simulink model "untitled"  (R2017b)
settings: Solver=VariableStepAuto  StartTime=0.0  StopTime=10.0  RelTol=1e-3
values from neighbouring files (symbols this model uses):
  Lst = 3/epsilonO2L    (= 12.9310344828)    [Lambda.m]
undefined symbols (not defined in the file or in its folder): mK
settings Model: Creator=irene  LastModifiedBy=irene

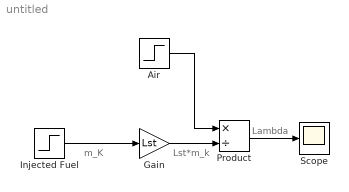
== system untitled ==
  note: Lst*m_k
  note: m_K
  note: Lambda
  "Air " : Step  SampleTime=0
  Gain : Gain  Gain=Lst
  Injected Fuel : Step  After=mK  SampleTime=0
  Product : Product  Inputs=*/  RndMeth=Nearest
  Scope : Scope
  wires:
  Injected Fuel/1 -> Gain/1
  Gain/1 -> Product/2
  "Air "/1 -> Product/1
  Product/1 -> Scope/1
